simulink model "Receiver_FPGACap"  (R2019b)
settings: Solver=FixedStepDiscrete  StartTime=0.0  StopTime=10.0  RelTol=1e-3
InitFcn:
  | modelSettings
undefined symbols (not defined in the file): crcDecodeLag, RadioSampleRate, VibertiTracebackLength
libraries: simulink x4, RxTxFixedPointLibrary_noscopes x2, dspsigops x2, commsource2 x1, hdlverifier_fpga_debug x1
settings Model: Creator=tcollins  LastModifiedBy=bhisma
settings DataIOCC: ReturnWorkspaceOutputs=off
settings OptimizationCC: BlockReduction=off  ConditionallyExecuteInputs=off  DefaultParameterBehavior=Inlined
settings DebuggingCC: AlgebraicLoopMsg=error  SingleTaskRateTransMsg=error  ArithmeticOperatorsInVariantConditions=warning
settings HardwareCC: ProdBitPerPointer=32  ProdBitPerSizeT=32  ProdBitPerPtrDiffT=32  ProdLargestAtomicFloat=None  ProdIntDivRoundTo=Undefined  ProdEndianess=Unspecified  ProdWordSize=32  ProdHWDeviceType=ASIC/FPGA->ASIC/FPGA  ProdEqTarget=off
settings SFSimCC: SimUseLocalCustomCode=off  CustomCodeUndefinedFunction=UseInterfaceOnly
settings RTWCC: RTWUseLocalCustomCode=off
settings CodeAppCC: StateflowObjectComments=on

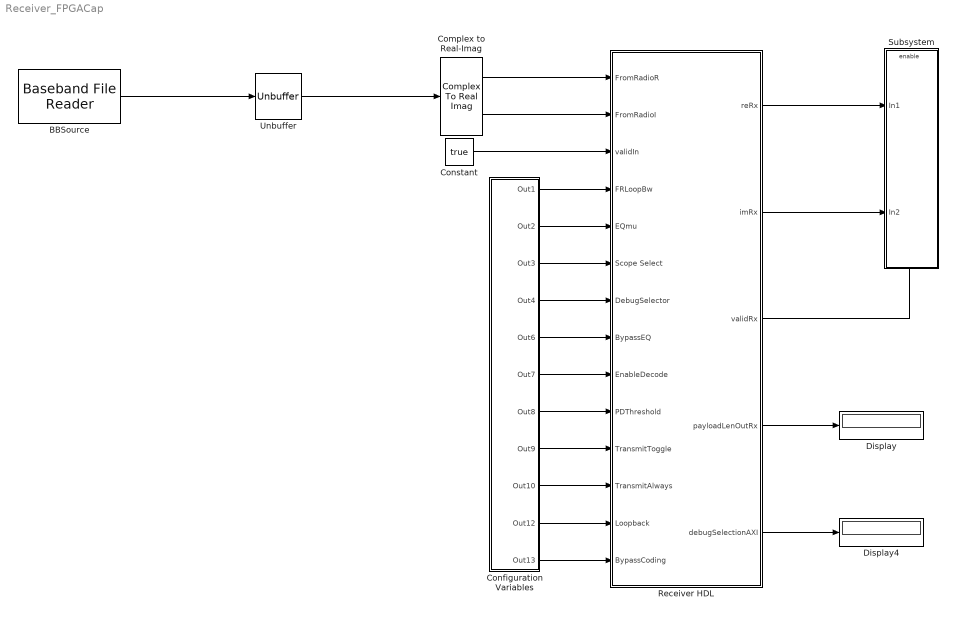
== system Receiver_FPGACap ==
  BBSource : commsource2/Baseband File Reader  Filename=CRCErrorData.bb  InheritSampleTimeFromFile=off  SampleTime=100000/(RadioSampleRate)  SamplesPerFrame=100000  CyclicRepetition=off  FileEndOutputPort=off  SimulateUsing=Interpreted execution
      settings: SourceProductName=Communications Toolbox  SourceProductBaseCode=CM
  Complex to Real-Imag : ComplexToRealImag
  Configuration Variables : Subsystem
  Constant : Constant  Value=true  SampleTime=-1
  Display : Display
  Display4 : Display
  Receiver HDL : Subsystem  TreatAsAtomicUnit=on
  Subsystem : Subsystem
  Unbuffer : Unbuffer
  wires:
  BBSource/1 -> Unbuffer/1
  Complex to Real-Imag/1 -> Receiver HDL/1(FromRadioR)
  Complex to Real-Imag/2 -> Receiver HDL/2(FromRadioI)
  Receiver HDL/3(validRx) -> Subsystem/Enable
  Configuration Variables/3(Out3) -> Receiver HDL/6(Scope Select)
  Configuration Variables/1(Out1) -> Receiver HDL/4(FRLoopBw)
  Configuration Variables/2(Out2) -> Receiver HDL/5(EQmu)
  Receiver HDL/5(debugSelectionAXI) -> Display4/1
  Configuration Variables/4(Out4) -> Receiver HDL/7(DebugSelector)
  Configuration Variables/5(Out6) -> Receiver HDL/8(BypassEQ)
  Configuration Variables/6(Out7) -> Receiver HDL/9(EnableDecode)
  Receiver HDL/4(payloadLenOutRx) -> Display/1
  Unbuffer/1 -> Complex to Real-Imag/1
  Configuration Variables/7(Out8) -> Receiver HDL/10(PDThreshold)
  Configuration Variables/8(Out9) -> Receiver HDL/11(TransmitToggle)
  Configuration Variables/9(Out10) -> Receiver HDL/12(TransmitAlways)
  Configuration Variables/10(Out12) -> Receiver HDL/13(Loopback)
  Configuration Variables/11(Out13) -> Receiver HDL/14(BypassCoding)
  Receiver HDL/1(reRx) -> Subsystem/1(In1)
  Receiver HDL/2(imRx) -> Subsystem/2(In2)
  Constant/1 -> Receiver HDL/3(validIn)

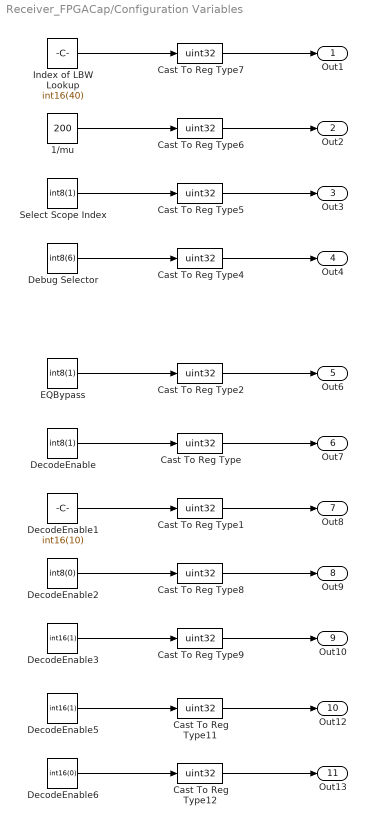
== system Receiver_FPGACap/Configuration Variables ==
  1/mu : Constant  Value=200  OutDataTypeStr=int16  SampleTime=-1
  Cast To Reg Type{,1..2,4..9,11..12} (11 alike) : DataTypeConversion  OutDataTypeStr=uint32
  Debug Selector : Constant  Value=int8(6)  SampleTime=1/RadioSampleRate
  DecodeEnable : Constant  Value=int8(1)  SampleTime=1/RadioSampleRate
  DecodeEnable1 : Constant  Value=int16(10)  SampleTime=1/RadioSampleRate
  DecodeEnable2 : Constant  Value=int8(0)  SampleTime=1/RadioSampleRate
  DecodeEnable3 : Constant  Value=int16(1)  SampleTime=1/RadioSampleRate
  DecodeEnable5 : Constant  Value=int16(1)  SampleTime=1/RadioSampleRate
  DecodeEnable6 : Constant  Value=int16(0)  SampleTime=1/RadioSampleRate
  EQBypass : Constant  Value=int8(1)  SampleTime=1/RadioSampleRate
  Index of LBW Lookup : Constant  Value=int16(40)  SampleTime=1/RadioSampleRate
  Select Scope Index : Constant  Value=int8(1)  SampleTime=1/RadioSampleRate
  Out1 : Outport  VectorParamsAs1DForOutWhenUnconnected=off
  Out2 : Outport  Port=2  VectorParamsAs1DForOutWhenUnconnected=off
  Out3 : Outport  Port=3  VectorParamsAs1DForOutWhenUnconnected=off
  Out4 : Outport  Port=4  VectorParamsAs1DForOutWhenUnconnected=off
  Out6 : Outport  Port=5  VectorParamsAs1DForOutWhenUnconnected=off
  Out7 : Outport  Port=6  VectorParamsAs1DForOutWhenUnconnected=off
  Out8 : Outport  Port=7  VectorParamsAs1DForOutWhenUnconnected=off
  Out9 : Outport  Port=8  VectorParamsAs1DForOutWhenUnconnected=off
  Out10 : Outport  Port=9  VectorParamsAs1DForOutWhenUnconnected=off
  Out12 : Outport  Port=10  VectorParamsAs1DForOutWhenUnconnected=off
  Out13 : Outport  Port=11  VectorParamsAs1DForOutWhenUnconnected=off
  wires:
  1/mu/1 -> Cast To Reg Type6/1
  Index of LBW Lookup/1 -> Cast To Reg Type7/1
  Select Scope Index/1 -> Cast To Reg Type5/1
  Debug Selector/1 -> Cast To Reg Type4/1
  EQBypass/1 -> Cast To Reg Type2/1
  DecodeEnable/1 -> Cast To Reg Type/1
  DecodeEnable1/1 -> Cast To Reg Type1/1
  Cast To Reg Type1/1 -> Out8/1
  Cast To Reg Type/1 -> Out7/1
  Cast To Reg Type2/1 -> Out6/1
  Cast To Reg Type4/1 -> Out4/1
  Cast To Reg Type5/1 -> Out3/1
  Cast To Reg Type6/1 -> Out2/1
  Cast To Reg Type7/1 -> Out1/1
  DecodeEnable2/1 -> Cast To Reg Type8/1
  DecodeEnable3/1 -> Cast To Reg Type9/1
  Cast To Reg Type9/1 -> Out10/1
  Cast To Reg Type8/1 -> Out9/1
  DecodeEnable5/1 -> Cast To Reg Type11/1
  Cast To Reg Type11/1 -> Out12/1
  DecodeEnable6/1 -> Cast To Reg Type12/1
  Cast To Reg Type12/1 -> Out13/1

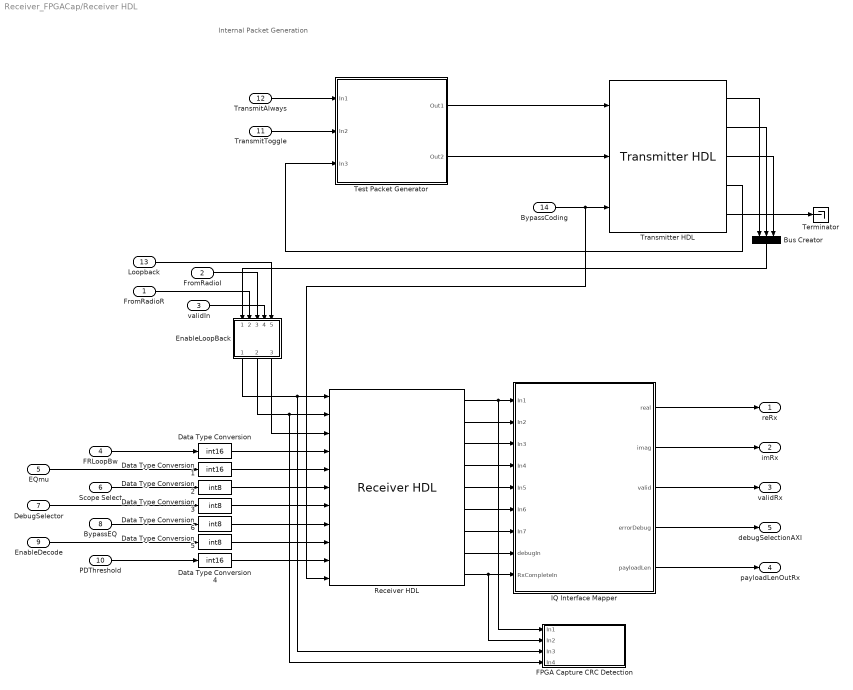
== system Receiver_FPGACap/Receiver HDL ==
  note: Internal Packet Generation
  FromRadioR : Inport
  FromRadioI : Inport  Port=2
  validIn : Inport  Port=3
  FRLoopBw : Inport  Port=4
  EQmu : Inport  Port=5
  Scope Select : Inport  Port=6
  DebugSelector : Inport  Port=7
  BypassEQ : Inport  Port=8
  EnableDecode : Inport  Port=9
  PDThreshold : Inport  Port=10
  TransmitToggle : Inport  Port=11
  TransmitAlways : Inport  Port=12
  Loopback : Inport  Port=13
  BypassCoding : Inport  Port=14
  Bus Creator : BusCreator  Inputs=3
  Data Type Conversion : DataTypeConversion  OutDataTypeStr=int16
  Data Type Conversion1 : DataTypeConversion  OutDataTypeStr=int16
  Data Type Conversion{2..3,5..6} (4 alike) : DataTypeConversion  OutDataTypeStr=int8
  Data Type Conversion4 : DataTypeConversion  OutDataTypeStr=int16
  EnableLoopBack : Subsystem
  FPGA Capture CRC Detection : Subsystem
  IQ Interface Mapper : Subsystem
  Receiver HDL : RxTxFixedPointLibrary_noscopes/Receiver HDL  SystemSampleTime=-1
  Terminator : Terminator
  Test Packet Generator : Subsystem
  Transmitter HDL : RxTxFixedPointLibrary_noscopes/Transmitter HDL  SystemSampleTime=-1
  reRx : Outport  VectorParamsAs1DForOutWhenUnconnected=off
  imRx : Outport  Port=2  VectorParamsAs1DForOutWhenUnconnected=off
  validRx : Outport  Port=3  VectorParamsAs1DForOutWhenUnconnected=off
  payloadLenOutRx : Outport  Port=4  VectorParamsAs1DForOutWhenUnconnected=off
  debugSelectionAXI : Outport  Port=5  VectorParamsAs1DForOutWhenUnconnected=off
  wires:
  Transmitter HDL/2 -> Bus Creator/2
  Transmitter HDL/3 -> Bus Creator/3
  Transmitter HDL/1 -> Bus Creator/1
  Transmitter HDL/4 -> Test Packet Generator/3(In3)
  FRLoopBw/1 -> Data Type Conversion/1
  EQmu/1 -> Data Type Conversion1/1
  Scope Select/1 -> Data Type Conversion2/1
  DebugSelector/1 -> Data Type Conversion3/1
  BypassEQ/1 -> Data Type Conversion6/1
  EnableDecode/1 -> Data Type Conversion5/1
  Receiver HDL/1 -> FPGA Capture CRC Detection/1(In1), IQ Interface Mapper/1(In1)
  Receiver HDL/2 -> IQ Interface Mapper/2(In2)
  Receiver HDL/3 -> IQ Interface Mapper/3(In3)
  Receiver HDL/4 -> IQ Interface Mapper/4(In4)
  Receiver HDL/5 -> IQ Interface Mapper/5(In5)
  Receiver HDL/6 -> IQ Interface Mapper/6(In6)
  Receiver HDL/7 -> IQ Interface Mapper/7(In7)
  IQ Interface Mapper/5(payloadLen) -> payloadLenOutRx/1
  IQ Interface Mapper/1(real) -> reRx/1
  IQ Interface Mapper/2(imag) -> imRx/1
  IQ Interface Mapper/3(valid) -> validRx/1
  IQ Interface Mapper/4(errorDebug) -> debugSelectionAXI/1
  Transmitter HDL/5 -> Terminator/1
  PDThreshold/1 -> Data Type Conversion4/1
  Data Type Conversion/1 -> Receiver HDL/4
  Data Type Conversion1/1 -> Receiver HDL/5
  Data Type Conversion2/1 -> Receiver HDL/6
  Data Type Conversion3/1 -> Receiver HDL/7
  Data Type Conversion4/1 -> Receiver HDL/10
  Data Type Conversion5/1 -> Receiver HDL/9
  Data Type Conversion6/1 -> Receiver HDL/8
  EnableLoopBack/1(Out1) -> FPGA Capture CRC Detection/3(In3), Receiver HDL/1
  EnableLoopBack/2(Out2) -> FPGA Capture CRC Detection/4(In4), Receiver HDL/2
  EnableLoopBack/3(Out3) -> Receiver HDL/3
  FromRadioR/1 -> EnableLoopBack/2(In1)
  FromRadioI/1 -> EnableLoopBack/3(In2)
  Bus Creator/1 -> EnableLoopBack/1(In5)
  validIn/1 -> EnableLoopBack/4(In3)
  Loopback/1 -> EnableLoopBack/5(In4)
  BypassCoding/1 -> Receiver HDL/11, Transmitter HDL/3
  TransmitAlways/1 -> Test Packet Generator/1(In1)
  TransmitToggle/1 -> Test Packet Generator/2(In2)
  Test Packet Generator/1(Out1) -> Transmitter HDL/1
  Test Packet Generator/2(Out2) -> Transmitter HDL/2
  Receiver HDL/8 -> IQ Interface Mapper/8(debugIn)
  Receiver HDL/9 -> FPGA Capture CRC Detection/2(In2), IQ Interface Mapper/9(RxCompleteIn)

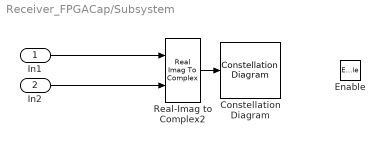
== system Receiver_FPGACap/Subsystem ==
  In1 : Inport
  In2 : Inport  Port=2
  Enable : EnablePort
  Constellation Diagram : ConstellationDiagram
  Real-Imag to Complex2 : RealImagToComplex
  wires:
  Real-Imag to Complex2/1 -> Constellation Diagram/1
  In1/1 -> Real-Imag to Complex2/1
  In2/1 -> Real-Imag to Complex2/2

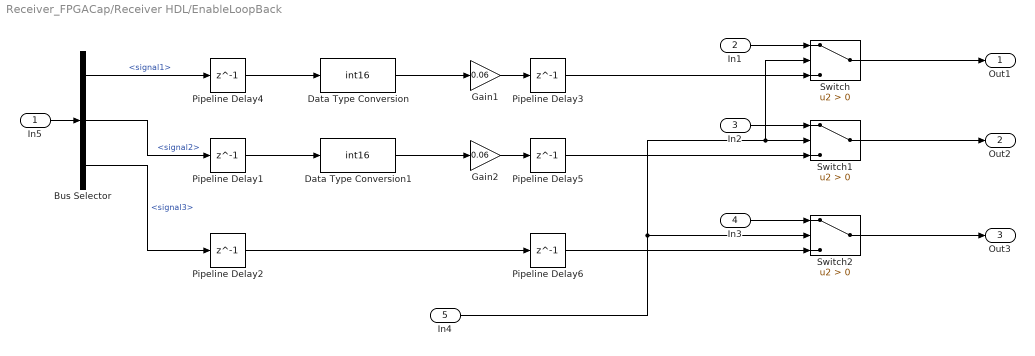
== system Receiver_FPGACap/Receiver HDL/EnableLoopBack ==
  In5 : Inport
  In1 : Inport  Port=2
  In2 : Inport  Port=3
  In3 : Inport  Port=4
  In4 : Inport  Port=5
  Bus Selector : BusSelector  OutputSignals=signal1,signal2,signal3
  Data Type Conversion : DataTypeConversion  OutDataTypeStr=int16  ConvertRealWorld=Stored Integer (SI)
  Data Type Conversion1 : DataTypeConversion  OutDataTypeStr=int16  ConvertRealWorld=Stored Integer (SI)
  Gain1 : Gain  Gain=0.06  OutDataTypeStr=int16  SaturateOnIntegerOverflow=on
  Gain2 : Gain  Gain=0.06  OutDataTypeStr=int16  SaturateOnIntegerOverflow=on
  Pipeline Delay{1..6} (6 alike) : Delay  DelayLength=1
  Switch : Switch  Criteria=u2 > Threshold
  Switch1 : Switch  Criteria=u2 > Threshold
  Switch2 : Switch  Criteria=u2 > Threshold
  Out1 : Outport  VectorParamsAs1DForOutWhenUnconnected=off
  Out2 : Outport  Port=2  VectorParamsAs1DForOutWhenUnconnected=off
  Out3 : Outport  Port=3  VectorParamsAs1DForOutWhenUnconnected=off
  wires:
  Switch1/1 -> Out2/1
  Switch2/1 -> Out3/1
  Switch/1 -> Out1/1
  In4/1 -> Switch/2, Switch1/2, Switch2/2
  Pipeline Delay4/1 -> Data Type Conversion/1
  Pipeline Delay1/1 -> Data Type Conversion1/1
  Pipeline Delay2/1 -> Pipeline Delay6/1
  In5/1 -> Bus Selector/1
  Bus Selector/1 -> Pipeline Delay4/1  "<signal1>"
  Bus Selector/2 -> Pipeline Delay1/1  "<signal2>"
  Bus Selector/3 -> Pipeline Delay2/1  "<signal3>"
  Data Type Conversion/1 -> Gain1/1
  Gain1/1 -> Pipeline Delay3/1
  Data Type Conversion1/1 -> Gain2/1
  Gain2/1 -> Pipeline Delay5/1
  In1/1 -> Switch/1
  Pipeline Delay3/1 -> Switch/3
  In2/1 -> Switch1/1
  Pipeline Delay5/1 -> Switch1/3
  In3/1 -> Switch2/1
  Pipeline Delay6/1 -> Switch2/3

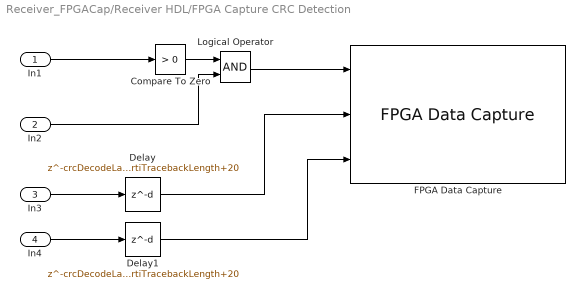
== system Receiver_FPGACap/Receiver HDL/FPGA Capture CRC Detection ==
  In1 : Inport
  In2 : Inport  Port=2
  In3 : Inport  Port=3
  In4 : Inport  Port=4
  Compare To Zero : simulink/Logic and Bit Operations/Compare To Zero  relop=>  OutDataTypeStr=boolean
  Delay : Delay  DelayLength=crcDecodeLag+VibertiTracebackLength+20
  Delay1 : Delay  DelayLength=crcDecodeLag+VibertiTracebackLength+20
  FPGA Data Capture : hdlverifier_fpga_debug/FPGA Data Capture  NumDataPorts=3  BufferSize=32768
      settings: SourceProductName=HDL Verifier Support Package for Xilinx FPGA Boards  SourceProductBaseCode=HDLCVXILINX
  Logical Operator : Logic  AllPortsSameDT=off  OutDataTypeStr=boolean
  wires:
  In3/1 -> Delay/1
  In4/1 -> Delay1/1
  Compare To Zero/1 -> Logical Operator/1
  In2/1 -> Logical Operator/2
  Logical Operator/1 -> FPGA Data Capture/1
  Delay/1 -> FPGA Data Capture/2
  In1/1 -> Compare To Zero/1
  Delay1/1 -> FPGA Data Capture/3

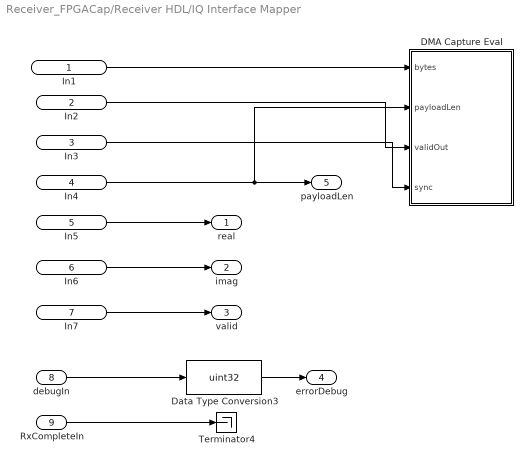
== system Receiver_FPGACap/Receiver HDL/IQ Interface Mapper ==
  In1 : Inport
  In2 : Inport  Port=2
  In3 : Inport  Port=3
  In4 : Inport  Port=4
  In5 : Inport  Port=5
  In6 : Inport  Port=6
  In7 : Inport  Port=7
  debugIn : Inport  Port=8
  RxCompleteIn : Inport  Port=9
  DMA Capture Eval : MATLAB Function  TreatAsAtomicUnit=on
  Data Type Conversion3 : DataTypeConversion  OutDataTypeStr=uint32
  Terminator4 : Terminator
  real : Outport  VectorParamsAs1DForOutWhenUnconnected=off
  imag : Outport  Port=2  VectorParamsAs1DForOutWhenUnconnected=off
  valid : Outport  Port=3  VectorParamsAs1DForOutWhenUnconnected=off
  errorDebug : Outport  Port=4  VectorParamsAs1DForOutWhenUnconnected=off
  payloadLen : Outport  Port=5  VectorParamsAs1DForOutWhenUnconnected=off
  wires:
  In2/1 -> DMA Capture Eval/3(validOut)
  In7/1 -> valid/1
  debugIn/1 -> Data Type Conversion3/1
  In1/1 -> DMA Capture Eval/1(bytes)
  In3/1 -> DMA Capture Eval/4(sync)
  In5/1 -> real/1
  In6/1 -> imag/1
  Data Type Conversion3/1 -> errorDebug/1
  RxCompleteIn/1 -> Terminator4/1
  In4/1 -> DMA Capture Eval/2(payloadLen), payloadLen/1

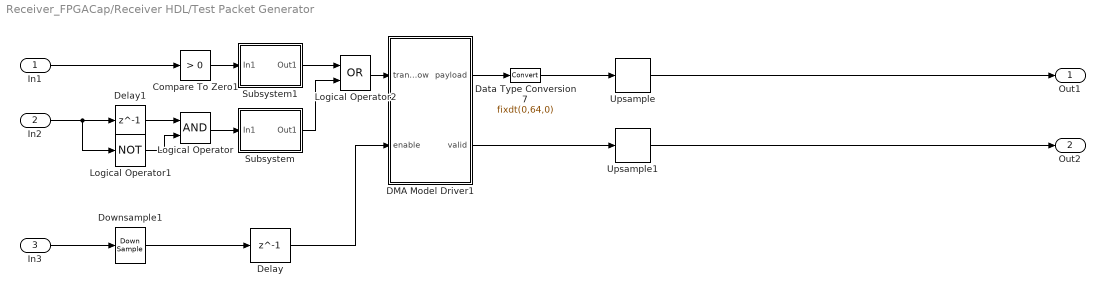
== system Receiver_FPGACap/Receiver HDL/Test Packet Generator ==
  In1 : Inport
  In2 : Inport  Port=2
  In3 : Inport  Port=3
  Compare To Zero1 : simulink/Logic and Bit Operations/Compare To Zero  relop=>  OutDataTypeStr=boolean
  DMA Model Driver1 : MATLAB Function  TreatAsAtomicUnit=on
  Data Type Conversion7 : DataTypeConversion  OutDataTypeStr=fixdt(0,64,0)
  Delay : Delay  DelayLength=1
  Delay1 : Delay  DelayLength=1
  Downsample1 : DownSample  N=4  RateOptions=Allow multirate processing
  Logical Operator : Logic  AllPortsSameDT=off  OutDataTypeStr=boolean
  Logical Operator1 : Logic  Operator=NOT  AllPortsSameDT=off  OutDataTypeStr=boolean
  Logical Operator2 : Logic  Operator=OR  AllPortsSameDT=off  OutDataTypeStr=boolean
  Subsystem : Subsystem
  Subsystem1 : Subsystem
  Upsample : dspsigops/Upsample  N=4  phase=0  RateOptions=Allow multirate processing  ic=0  mode=Unused parameter value
  Upsample1 : dspsigops/Upsample  N=4  phase=0  RateOptions=Allow multirate processing  ic=0  mode=Unused parameter value
  Out1 : Outport  VectorParamsAs1DForOutWhenUnconnected=off
  Out2 : Outport  Port=2  VectorParamsAs1DForOutWhenUnconnected=off
  wires:
  In1/1 -> Compare To Zero1/1
  Subsystem/1(Out1) -> Logical Operator2/2
  Logical Operator1/1 -> Logical Operator/2
  DMA Model Driver1/1(payload) -> Data Type Conversion7/1
  Downsample1/1 -> Delay/1
  Delay1/1 -> Logical Operator/1
  Logical Operator/1 -> Subsystem/1(In1)
  Logical Operator2/1 -> DMA Model Driver1/1(transmitNow)
  Subsystem1/1(Out1) -> Logical Operator2/1
  In2/1 -> Logical Operator1/1, Delay1/1
  DMA Model Driver1/2(valid) -> Upsample1/1
  Data Type Conversion7/1 -> Upsample/1
  Compare To Zero1/1 -> Subsystem1/1(In1)
  Upsample1/1 -> Out2/1
  Upsample/1 -> Out1/1
  Delay/1 -> DMA Model Driver1/2(enable)
  In3/1 -> Downsample1/1

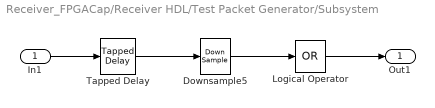
== system Receiver_FPGACap/Receiver HDL/Test Packet Generator/Subsystem ==
  In1 : Inport
  Downsample5 : DownSample  N=4  RateOptions=Allow multirate processing
  Logical Operator : Logic  Operator=OR  Inputs=1  AllPortsSameDT=off  OutDataTypeStr=boolean
  Tapped Delay : simulink/Discrete/Tapped Delay  vinit=0.0  samptime=-1  NumDelays=3  DelayOrder=Oldest  includeCurrent=on
  Out1 : Outport  VectorParamsAs1DForOutWhenUnconnected=off
  wires:
  Logical Operator/1 -> Out1/1
  Downsample5/1 -> Logical Operator/1
  Tapped Delay/1 -> Downsample5/1
  In1/1 -> Tapped Delay/1

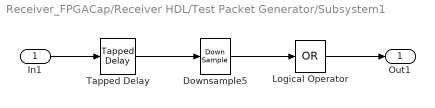
== system Receiver_FPGACap/Receiver HDL/Test Packet Generator/Subsystem1 ==
  In1 : Inport
  Downsample5 : DownSample  N=4  RateOptions=Allow multirate processing
  Logical Operator : Logic  Operator=OR  Inputs=1  AllPortsSameDT=off  OutDataTypeStr=boolean
  Tapped Delay : simulink/Discrete/Tapped Delay  vinit=0.0  samptime=-1  NumDelays=3  DelayOrder=Oldest  includeCurrent=on
  Out1 : Outport  VectorParamsAs1DForOutWhenUnconnected=off
  wires:
  Logical Operator/1 -> Out1/1
  Downsample5/1 -> Logical Operator/1
  Tapped Delay/1 -> Downsample5/1
  In1/1 -> Tapped Delay/1

== matlab function Receiver_FPGACap/Receiver HDL/IQ Interface Mapper/DMA Capture Eval ==
  data: bytes input; payloadLen input; validOut input; sync input
function fcn(bytes, payloadLen, validOut, sync)

persistent frameBuffer byteCounter fullPayloadBits

bitsInPack = 64;

if isempty(frameBuffer)
    maxFrameBits = (2^16)*8;
    frameBuffer = false(maxFrameBits,1);
    byteCounter = 0;
    fullPayloadBits = uint16(0);
end

if validOut
    if sync
        byteCounter = bitsInPack;
        frameBuffer(1:byteCounter) = bitget(bytes,1:bitsInPack);
        fullPayloadBits = uint16(payloadLen*8);
        
    elseif byteCounter<fullPayloadBits
        frameBuffer(byteCounter+1:byteCounter+bitsInPack) = bitget(bytes,1:bitsInPack);
        byteCounter = byteCounter + bitsInPack;
    else
        if bytes>0
            disp('CRC Error (Outside)');
            ref = load('bits.mat');
            bref = ref.bits(1:end-32);
            b = frameBuffer(1:byteCounter);
            wrongBitPosition = find(bref~=b);
            fprintf('Wrong bit positions: ');
            for k=1:length(wrongBitPosition)
                fprintf('%d ',int16(wrongBitPosition(k)));
            end
            fprintf('\n');
        else
            disp('Frame passed CRC (Outside)');
            b = frameBuffer(1:byteCounter);
            fprintf('%s\n',char(bi2de(reshape(b,64,832/64).').'));
        end
    end
end

== matlab function Receiver_FPGACap/Receiver HDL/Test Packet Generator/DMA Model Driver1 ==
  data: transmitNow input; payload output; valid output boolean; enable input
function [payload,valid] = fcn(transmitNow, enable)
%#codegen

persistent indx mode pSize counter msg payloadIndx transmitNext

if isempty(indx)
    msg = fi(int8('Hello World 0'),0,64,0);
    pSize = fi(length('Hello World 0')*8,0,64,0); % Size in bytes (Must be multiple of 32 bits) cannot exceed uint16 max
    indx = pSize;
    mode = int8(0);
    counter = fi(0,0,64,0);
    payloadIndx = uint8(0);
    transmitNext = false;
end

%% Make default MSG
% Constant

% Update packet count
%msg(uint8(13)) = counter + fi(48,0,64,0);
setting = pSize;

%% Output MSG
if enable
    valid = true;
    switch mode
        case int8(0) % Fresh packet start
            if transmitNow || transmitNext
                pSize = fi(setting,0,64,0);
                payload = fi(setting,0,64,0);%Upper bits
                mode = int8(1);
                payloadIndx = uint8(0);
                indx = fi(0,0,64,0);
                transmitNext = false; % Reset
                %fprintf('(TX) Sending new packet with length: %u\n',uint64(pSize));
            else
                payload = fi(setting,0,64,0);%Upper bits
                valid = false;
            end
        otherwise
            if transmitNow
                transmitNext = true;
            end
            indx = fi(indx + fi(8,0,64,0),0,64,0);
            payloadIndx = payloadIndx + uint8(1);
            payload = msg(payloadIndx);
            if indx == pSize % reached end of frame
                mode = int8(0);
                payloadIndx = uint8(0);
                if counter==fi(9,0,64,0)
                    counter = fi(0,0,64,0);
                else
                    counter = fi(counter + fi(1,0,64,0),0,64,0);
                end
            end
    end
else
    if transmitNow
        transmitNext = true;
    end
    valid = false;
    payload = fi(0,0,64,0);
end
